simulink model "Filter1simulink1"  (R2019b)
settings: Solver=VariableStepAuto  StartTime=0.0  StopTime=10.0  RelTol=1e-3
settings Model: Creator=pahul  LastModifiedBy=pahul

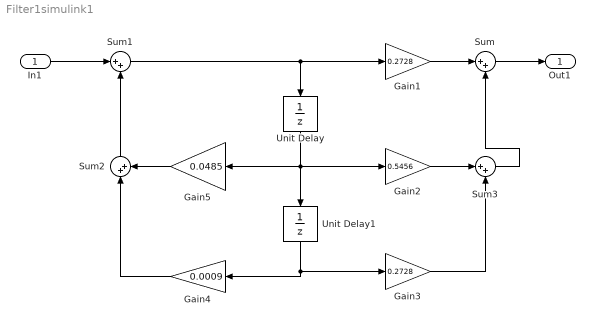
== system Filter1simulink1 ==
  In1 : Inport
  Gain1 : Gain  Gain=0.2728
  Gain2 : Gain  Gain=0.5456
  Gain3 : Gain  Gain=0.2728
  Gain4 : Gain  Gain=0.0009
  Gain5 : Gain  Gain=0.0485
  Sum{,1..3} (4 alike) : Sum  Inputs=|++
  Unit Delay : UnitDelay  SampleTime=-1  HasFrameUpgradeWarning=on
  Unit Delay1 : UnitDelay  SampleTime=-1  HasFrameUpgradeWarning=on
  Out1 : Outport
  wires:
  Unit Delay1/1 -> Gain3/1, Gain4/1
  Gain1/1 -> Sum/1
  Gain2/1 -> Sum3/1
  Gain3/1 -> Sum3/2
  Sum3/1 -> Sum/2
  In1/1 -> Sum1/1
  Sum1/1 -> Gain1/1, Unit Delay/1
  Sum/1 -> Out1/1
  Gain4/1 -> Sum2/1
  Unit Delay/1 -> Unit Delay1/1, Gain5/1, Gain2/1
  Gain5/1 -> Sum2/2
  Sum2/1 -> Sum1/2
